simulink model "AGTF30SysDyn_PExPIn"  (R2021b)
settings: Solver=ode4  StartTime=0.0  StopTime=MWS.In.tend  FixedStep=MWS.In.Ts  RelTol=1e-3  EnableMultiTasking=on
model workspace: external: MAT-File (data not in the file)
values from neighbouring files (symbols this model uses):
  MWS = setup_initialize(MWS,startPt,SSsolverSP)    [Setup_Simulation.m]    (also in run_AGTF30e_script.m = Setup_Simulation(inputMethod,MWS.In,filename,Mdl,SSsolverSP,)
undefined symbols (not defined in the file or in its folder): DiscIntNeverNeededParam
libraries: Lib_Solve_ModelSource_TMATS x28, Lib_Cntrl_FirstOrderSensor_TMATS x19, simulink x12, Lib_Cntrl_FirstOrderActuator_TMATS x2, Lib_Cntrl_LimitSelect_TMATS x2, Lib_Solve_OuterLoopIntegrator_TMATS x2, Lib_Cntrl_CorrectedSpeed_TMATS x1, Lib_Solve_IterNRSolverJC_TMATS x1
(part 6 of 6)

== system AGTF30SysDyn_PExPIn/Control System/Scheduling/Steady State EM Power - MaxMin/HP and LP Pwr Calc/Gearbox Speeds/Spool to PGB speeds ==
  note: Sun
      | Ring
      | Carrier
  note: Sun
      | Ring
      | Carrier
  N : Inport
  Constant : Constant  Value=MWS.In.Options.PGBConfig
  Demux1 : Demux  Outputs=2
  Epicyclic Gearbox Speed Calc - RC : Subsystem  mask(Epicyclic Gearbox Speed Calc - SC){rS_M=MWS.Shaft.PGB.Sun.r, rR_M=MWS.Shaft.PGB.Ring.r}
      mask prompts: rS_M "rS_M - Sun gear radius, ft"; rR_M "rR_M - Ring gear radius, ft"
      mask help: This block outputs the rotational speeds of all 4 epicyclic gearbox components (sun, ring, carrier, planets) given the speeds of the sun gear and carrier. Units are consistent with input units.
      mask init:
      | rP_I = 0.5*(rR_M-rS_M);
  Epicyclic Gearbox Speed Calc - RC1 : Subsystem  mask(Epicyclic Gearbox Speed Calc - SC){rS_M=MWS.Shaft.PGB.Sun.r, rR_M=MWS.Shaft.PGB.Ring.r}
      mask prompts: rS_M "rS_M - Sun gear radius, ft"; rR_M "rR_M - Ring gear radius, ft"
      mask help: This block outputs the rotational speeds of all 4 epicyclic gearbox components (sun, ring, carrier, planets) given the speeds of the sun gear and carrier. Units are consistent with input units.
      mask init:
      | rP_I = 0.5*(rR_M-rS_M);
  Epicyclic Gearbox Speed Calc - SC : Subsystem  mask(Epicyclic Gearbox Speed Calc - SC){rS_M=MWS.Shaft.PGB.Sun.r, rR_M=MWS.Shaft.PGB.Ring.r}
      mask prompts: rS_M "rS_M - Sun gear radius, ft"; rR_M "rR_M - Ring gear radius, ft"
      mask help: This block outputs the rotational speeds of all 4 epicyclic gearbox components (sun, ring, carrier, planets) given the speeds of the sun gear and carrier. Units are consistent with input units.
      mask init:
      | rP_I = 0.5*(rR_M-rS_M);
  Epicyclic Gearbox Speed Calc - SC1 : Subsystem  mask(Epicyclic Gearbox Speed Calc - SC){rS_M=MWS.Shaft.PGB.Sun.r, rR_M=MWS.Shaft.PGB.Ring.r}
      mask prompts: rS_M "rS_M - Sun gear radius, ft"; rR_M "rR_M - Ring gear radius, ft"
      mask help: This block outputs the rotational speeds of all 4 epicyclic gearbox components (sun, ring, carrier, planets) given the speeds of the sun gear and carrier. Units are consistent with input units.
      mask init:
      | rP_I = 0.5*(rR_M-rS_M);
  Epicyclic Gearbox Speed Calc - SR : Subsystem  mask(Epicyclic Gearbox Speed Calc - SR){rS_M=MWS.Shaft.PGB.Sun.r, rR_M=MWS.Shaft.PGB.Ring.r}
      mask prompts: rS_M "rS_M - Radius of the sun gear, ft"; rR_M "rR_M - Radius of the ring gear, ft"
      mask help: This block outputs the rotational speeds of all 4 epicyclic gearbox components (sun, ring, carrier, planets) given the speeds of the sun gear and ring gear. Units are consistent with input units.
      mask init:
      | rP_I = 0.5*(rR_M-rS_M);
  Epicyclic Gearbox Speed Calc - SR1 : Subsystem  mask(Epicyclic Gearbox Speed Calc - SR){rS_M=MWS.Shaft.PGB.Sun.r, rR_M=MWS.Shaft.PGB.Ring.r}
      mask prompts: rS_M "rS_M - Radius of the sun gear, ft"; rR_M "rR_M - Radius of the ring gear, ft"
      mask help: This block outputs the rotational speeds of all 4 epicyclic gearbox components (sun, ring, carrier, planets) given the speeds of the sun gear and ring gear. Units are consistent with input units.
      mask init:
      | rP_I = 0.5*(rR_M-rS_M);
  Gain1 : Gain  Gain=MWS.Shaft.PGB.Sun.GR_gb %GR = Ngb/Nint
  Gain19 : Gain  Gain=MWS.Shaft.PGB.Ring.GR_gb %GR = Ngb/Nint
  Gain2 : Gain  Gain=MWS.Shaft.PGB.Sun.GR_int %GR = Nint/Ncomp
  Gain20 : Gain  Gain=MWS.Shaft.PGB.Carrier.GR_int %GR = Nint/Ncomp
  Gain21 : Gain  Gain=MWS.Shaft.PGB.Carrier.GR_gb %GR = Ngb/Nint
  Gain22 : Gain  Gain=MWS.Shaft.PGB.Ring.GR_int %GR = Nint/Ncomp
  Gain23 : Gain  Gain=MWS.Shaft.PGB.Sun.GR_gb %GR = Ngb/Nint
  Gain24 : Gain  Gain=MWS.Shaft.PGB.Ring.GR_gb %GR = Ngb/Nint
  Gain25 : Gain  Gain=MWS.Shaft.PGB.Sun.GR_int %GR = Nint/Ncomp
  Gain26 : Gain  Gain=MWS.Shaft.PGB.Carrier.GR_int %GR = Nint/Ncomp
  Gain27 : Gain  Gain=MWS.Shaft.PGB.Carrier.GR_gb %GR = Ngb/Nint
  Gain28 : Gain  Gain=MWS.Shaft.PGB.Ring.GR_int %GR = Nint/Ncomp
  Multiport Switch2 : MultiPortSwitch  Inputs=6
  NPGB : Outport
  wires:
  Demux1/1 -> Gain20/1, Gain22/1, Gain2/1  "N2"
  Gain27/1 -> [NC_HP]
  Epicyclic Gearbox Speed Calc - RC1/1(N) -> Multiport Switch2/7
  Epicyclic Gearbox Speed Calc - SR1/1(N) -> Multiport Switch2/4
  Gain22/1 -> Gain19/1
  [NS_LP] -> Epicyclic Gearbox Speed Calc - SR1/1(NS)
  [NR_LP] -> Epicyclic Gearbox Speed Calc - RC1/1(NR)
  N/1 -> Demux1/1
  Gain20/1 -> Gain21/1
  Gain28/1 -> Gain24/1
  [NC_LP] -> Epicyclic Gearbox Speed Calc - SC/2(NC)
  Gain2/1 -> Gain1/1
  [NS_HP] -> Epicyclic Gearbox Speed Calc - SC/1(NS)
  Multiport Switch2/1 -> NPGB/1
  [NR_LP] -> Epicyclic Gearbox Speed Calc - SR/2(NR)
  Gain24/1 -> [NR_HP]
  [NR_HP] -> Epicyclic Gearbox Speed Calc - RC/1(NR)
  Demux1/2 -> Gain26/1, Gain28/1, Gain25/1  "N3"
  Gain26/1 -> Gain27/1
  Gain25/1 -> Gain23/1
  Gain1/1 -> [NS_LP]
  Epicyclic Gearbox Speed Calc - SC/1(N) -> Multiport Switch2/3
  [NS_HP] -> Epicyclic Gearbox Speed Calc - SR/1(NS)
  Gain19/1 -> [NR_LP]
  Gain21/1 -> [NC_LP]
  Gain23/1 -> [NS_HP]
  Epicyclic Gearbox Speed Calc - SR/1(N) -> Multiport Switch2/2
  [NC_HP] -> Epicyclic Gearbox Speed Calc - SC1/2(NC)
  [NC_HP] -> Epicyclic Gearbox Speed Calc - RC1/2(NC)
  [NS_LP] -> Epicyclic Gearbox Speed Calc - SC1/1(NS)
  Epicyclic Gearbox Speed Calc - RC/1(N) -> Multiport Switch2/5
  Constant/1 -> Multiport Switch2/1
  [NR_HP] -> Epicyclic Gearbox Speed Calc - SR1/2(NR)
  [NC_LP] -> Epicyclic Gearbox Speed Calc - RC/2(NC)
  Epicyclic Gearbox Speed Calc - SC1/1(N) -> Multiport Switch2/6

== system AGTF30SysDyn_PExPIn/Control System/Scheduling/Steady State EM Power - MaxMin/HP and LP Pwr Calc/Gearbox Speeds/Spool to PGB speeds/Epicyclic Gearbox Speed Calc - RC ==
  NR : Inport
  NC : Inport  Port=2
  Gain1 : Gain  Gain=rP_I
  Gain2 : Gain  Gain=rS_M
  Gain30 : Gain  Gain=rR_M/rP_I
  Gain31 : Gain  Gain=1/rS_M
  Mux4 : Mux
  Sum : Sum  Inputs=|+-
  Sum2 : Sum  Inputs=|+-
  N : Outport
  wires:
  NC/1 -> Gain2/1, Mux4/3, Sum/2  "NC"
  NR/1 -> Mux4/2, Sum/1  "NR"
  Mux4/1 -> N/1
  Sum/1 -> Gain30/1
  Gain30/1 -> Mux4/4, Gain1/1  "NP"
  Gain1/1 -> Sum2/2
  Gain2/1 -> Sum2/1
  Sum2/1 -> Gain31/1
  Gain31/1 -> Mux4/1  "NS"

== system AGTF30SysDyn_PExPIn/Control System/Scheduling/Steady State EM Power - MaxMin/HP and LP Pwr Calc/Gearbox Speeds/Spool to PGB speeds/Epicyclic Gearbox Speed Calc - RC1 ==
  NR : Inport
  NC : Inport  Port=2
  Gain1 : Gain  Gain=rP_I
  Gain2 : Gain  Gain=rS_M
  Gain30 : Gain  Gain=rR_M/rP_I
  Gain31 : Gain  Gain=1/rS_M
  Mux4 : Mux
  Sum : Sum  Inputs=|+-
  Sum2 : Sum  Inputs=|+-
  N : Outport
  wires:
  Gain31/1 -> Mux4/1  "NS"
  Sum2/1 -> Gain31/1
  Gain2/1 -> Sum2/1
  Gain1/1 -> Sum2/2
  Gain30/1 -> Gain1/1, Mux4/4  "NP"
  Sum/1 -> Gain30/1
  Mux4/1 -> N/1
  NR/1 -> Sum/1, Mux4/2  "NR"
  NC/1 -> Sum/2, Mux4/3, Gain2/1  "NC"

== system AGTF30SysDyn_PExPIn/Control System/Scheduling/Steady State EM Power - MaxMin/HP and LP Pwr Calc/Gearbox Speeds/Spool to PGB speeds/Epicyclic Gearbox Speed Calc - SC ==
  NS : Inport
  NC : Inport  Port=2
  Gain1 : Gain  Gain=rP_I
  Gain2 : Gain  Gain=rR_M
  Gain30 : Gain  Gain=rS_M/rP_I
  Gain31 : Gain  Gain=1/rR_M
  Mux4 : Mux
  Sum : Sum  Inputs=|-+
  Sum1 : Sum  Inputs=|++
  N : Outport
  wires:
  Mux4/1 -> N/1
  Gain31/1 -> Mux4/2  "NR"
  Gain30/1 -> Mux4/4, Gain1/1  "NP"
  NS/1 -> Sum/1, Mux4/1  "NS"
  Sum1/1 -> Gain31/1
  NC/1 -> Gain2/1, Mux4/3, Sum/2  "NC"
  Sum/1 -> Gain30/1
  Gain1/1 -> Sum1/1
  Gain2/1 -> Sum1/2

== system AGTF30SysDyn_PExPIn/Control System/Scheduling/Steady State EM Power - MaxMin/HP and LP Pwr Calc/Gearbox Speeds/Spool to PGB speeds/Epicyclic Gearbox Speed Calc - SC1 ==
  NS : Inport
  NC : Inport  Port=2
  Gain1 : Gain  Gain=rP_I
  Gain2 : Gain  Gain=rR_M
  Gain30 : Gain  Gain=rS_M/rP_I
  Gain31 : Gain  Gain=1/rR_M
  Mux4 : Mux
  Sum : Sum  Inputs=|-+
  Sum1 : Sum  Inputs=|++
  N : Outport
  wires:
  Gain2/1 -> Sum1/2
  Gain1/1 -> Sum1/1
  Sum/1 -> Gain30/1
  NC/1 -> Sum/2, Mux4/3, Gain2/1  "NC"
  Sum1/1 -> Gain31/1
  NS/1 -> Mux4/1, Sum/1  "NS"
  Gain30/1 -> Gain1/1, Mux4/4  "NP"
  Gain31/1 -> Mux4/2  "NR"
  Mux4/1 -> N/1

== system AGTF30SysDyn_PExPIn/Control System/Scheduling/Steady State EM Power - MaxMin/HP and LP Pwr Calc/Gearbox Speeds/Spool to PGB speeds/Epicyclic Gearbox Speed Calc - SR ==
  NS : Inport
  NR : Inport  Port=2
  Gain : Gain  Gain=rS_M
  Gain29 : Gain  Gain=rR_M
  Gain30 : Gain  Gain=1/(rS_M+rR_M)
  Gain31 : Gain  Gain=rS_M/rP_I
  Mux4 : Mux
  Sum : Sum  Inputs=|++
  Sum1 : Sum  Inputs=-+|
  N : Outport
  wires:
  NS/1 -> Mux4/1, Mux4/3, Sum1/1, Gain/1
  Sum/1 -> Gain30/1
  Gain29/1 -> Sum/2
  NR/1 -> Mux4/2, Gain29/1
  Sum1/1 -> Gain31/1
  Gain/1 -> Sum/1
  Gain30/1 -> Sum1/2  "NC"
  Gain31/1 -> Mux4/4  "NP"
  Mux4/1 -> N/1

== system AGTF30SysDyn_PExPIn/Control System/Scheduling/Steady State EM Power - MaxMin/HP and LP Pwr Calc/Gearbox Speeds/Spool to PGB speeds/Epicyclic Gearbox Speed Calc - SR1 ==
  NS : Inport
  NR : Inport  Port=2
  Gain : Gain  Gain=rS_M
  Gain29 : Gain  Gain=rR_M
  Gain30 : Gain  Gain=1/(rS_M+rR_M)
  Gain31 : Gain  Gain=rS_M/rP_I
  Mux4 : Mux
  Sum : Sum  Inputs=|++
  Sum1 : Sum  Inputs=-+|
  N : Outport
  wires:
  Mux4/1 -> N/1
  Gain31/1 -> Mux4/4  "NP"
  Gain30/1 -> Sum1/2  "NC"
  Gain/1 -> Sum/1
  Sum1/1 -> Gain31/1
  NR/1 -> Gain29/1, Mux4/2
  Gain29/1 -> Sum/2
  Sum/1 -> Gain30/1
  NS/1 -> Gain/1, Sum1/1, Mux4/3, Mux4/1

== matlab function AGTF30SysDyn_PExPIn/Actuators/LPS Electric Machine/Rate Limit Enforcement ==
  data: M_preRL input; M_act output; M_old input; Mdot_low input; Mdot_hi input; dt input
function M_act  = fcn(M_preRL,M_old,Mdot_low,Mdot_hi,dt)

M_act = M_preRL;
if (M_preRL < 0 && M_old > 0) || (M_preRL > 0 && M_old < 0)
    M_act = 0;
elseif M_preRL >= 0
    if (M_preRL-M_old)/dt > Mdot_hi
        M_act = M_old + Mdot_hi*dt;
    else
        M_act = M_preRL;
    end
elseif M_preRL < 0
    if (M_preRL-M_old)/dt < Mdot_low
        M_act = M_old + Mdot_low*dt;
    else
        M_act = M_preRL;
    end
end

== matlab function AGTF30SysDyn_PExPIn/Actuators/HPS Electric Machine/Rate Limit Enforcement ==
  data: M_preRL input; M_act output; M_old input; Mdot_low input; Mdot_hi input; dt input
function M_act  = fcn(M_preRL,M_old,Mdot_low,Mdot_hi,dt)

M_act = M_preRL;
if (M_preRL < 0 && M_old > 0) || (M_preRL > 0 && M_old < 0)
    M_act = 0;
elseif M_preRL >= 0
    if (M_preRL-M_old)/dt > Mdot_hi
        M_act = M_old + Mdot_hi*dt;
    else
        M_act = M_preRL;
    end
elseif M_preRL < 0
    if (M_preRL-M_old)/dt < Mdot_low
        M_act = M_old + Mdot_low*dt;
    else
        M_act = M_preRL;
    end
end

== matlab function AGTF30SysDyn_PExPIn/Actuators/Sun Gear Electric Machine/Rate Limit Enforcement ==
  data: M_preRL input; M_act output; M_old input; Mdot_low input; Mdot_hi input; dt input
function M_act  = fcn(M_preRL,M_old,Mdot_low,Mdot_hi,dt)

M_act = M_preRL;
if (M_preRL < 0 && M_old > 0) || (M_preRL > 0 && M_old < 0)
    M_act = 0;
elseif M_preRL >= 0
    if (M_preRL-M_old)/dt > Mdot_hi
        M_act = M_old + Mdot_hi*dt;
    else
        M_act = M_preRL;
    end
elseif M_preRL < 0
    if (M_preRL-M_old)/dt < Mdot_low
        M_act = M_old + Mdot_low*dt;
    else
        M_act = M_preRL;
    end
end

== matlab function AGTF30SysDyn_PExPIn/Actuators/Ring Gear Electric Machine/Rate Limit Enforcement ==
  data: M_preRL input; M_act output; M_old input; Mdot_low input; Mdot_hi input; dt input
function M_act  = fcn(M_preRL,M_old,Mdot_low,Mdot_hi,dt)

M_act = M_preRL;
if (M_preRL < 0 && M_old > 0) || (M_preRL > 0 && M_old < 0)
    M_act = 0;
elseif M_preRL >= 0
    if (M_preRL-M_old)/dt > Mdot_hi
        M_act = M_old + Mdot_hi*dt;
    else
        M_act = M_preRL;
    end
elseif M_preRL < 0
    if (M_preRL-M_old)/dt < Mdot_low
        M_act = M_old + Mdot_low*dt;
    else
        M_act = M_preRL;
    end
end

== matlab function AGTF30SysDyn_PExPIn/Actuators/Carrier Electric Machine/Rate Limit Enforcement ==
  data: M_preRL input; M_act output; M_old input; Mdot_low input; Mdot_hi input; dt input
function M_act  = fcn(M_preRL,M_old,Mdot_low,Mdot_hi,dt)

M_act = M_preRL;
if (M_preRL < 0 && M_old > 0) || (M_preRL > 0 && M_old < 0)
    M_act = 0;
elseif M_preRL >= 0
    if (M_preRL-M_old)/dt > Mdot_hi
        M_act = M_old + Mdot_hi*dt;
    else
        M_act = M_preRL;
    end
elseif M_preRL < 0
    if (M_preRL-M_old)/dt < Mdot_low
        M_act = M_old + Mdot_low*dt;
    else
        M_act = M_preRL;
    end
end

== matlab function AGTF30SysDyn_PExPIn/Actuators/Planet Gear Electric Machine/Rate Limit Enforcement ==
  data: M_preRL input; M_act output; M_old input; Mdot_low input; Mdot_hi input; dt input
function M_act  = fcn(M_preRL,M_old,Mdot_low,Mdot_hi,dt)

M_act = M_preRL;
if (M_preRL < 0 && M_old > 0) || (M_preRL > 0 && M_old < 0)
    M_act = 0;
elseif M_preRL >= 0
    if (M_preRL-M_old)/dt > Mdot_hi
        M_act = M_old + Mdot_hi*dt;
    else
        M_act = M_preRL;
    end
elseif M_preRL < 0
    if (M_preRL-M_old)/dt < Mdot_low
        M_act = M_old + Mdot_low*dt;
    else
        M_act = M_preRL;
    end
end
